simulink library "sm_testrig_common_gear_lib"  (R2021b)
settings: Solver=VariableStepAuto  StartTime=0.0  StopTime=10.0  RelTol=1e-3
values from neighbouring files (symbols this model uses):
  N = 10    [sm_extr_data_gear.m]
undefined symbols (not defined in the file or in its folder): b_gear_pd_asy, b_visc_frict_asy, f_gear_ad, f_gear_clr, f_gear_dd, f_gear_nt, f_gear_pd_asy, f_gear_rho, f_gear_rht, f_gear_th, f_mark_angle_range, f_mark_color, f_mark_radius_range, f_visc_frict_asy, X, Y, Z
libraries: sm_lib x8
settings Model: Creator=The MathWorks, Inc.  LastModifiedBy=The MathWorks, Inc.
settings SolverCC: AlgebraicLoopSolver=TrustRegion
settings DataIOCC: ReturnWorkspaceOutputs=off
settings DebuggingCC: SFMachineParentedDataDiag=warning  ArithmeticOperatorsInVariantConditions=warning
settings SFSimCC: SimUseLocalCustomCode=off  CustomCodeUndefinedFunction=UseInterfaceOnly
settings RTWCC: RTWUseLocalCustomCode=off

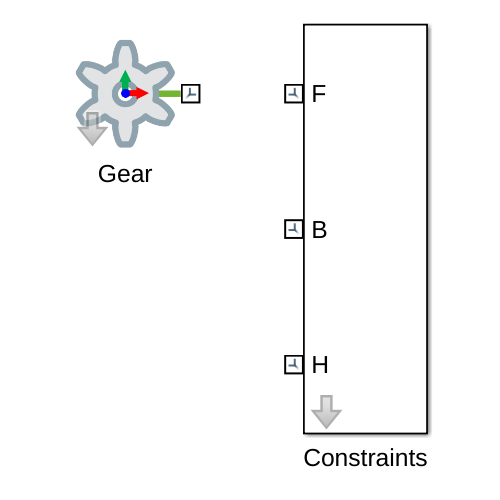
[thumbnail: Simulink's stored preview of the top-level diagram]
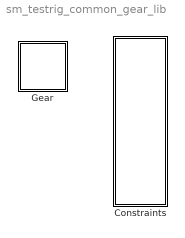
== system sm_testrig_common_gear_lib ==
  Constraints : Subsystem  mask(Common Gear Assembly Constraints){popup_gear_type=External, b_gear_pd=b_gear_pd_asy, f_gear_pd=f_gear_pd_asy, b_visc_frict=b_visc_frict_asy, f_visc_frict=f_visc_frict_asy}
      mask prompts: popup_gear_type "Gear Type"
      mask help: Model connects all required constraints for a common gear assembly. Contains two Revolute Joints and a Common Gear Constraint, all oriented and positioned according to the Common Gear Constraint requirements.
      mask init:
      | gear_constr_type = get_param(gcb,'popup_gear_type');
      | set_param([gcb '/Common Gear Constraint'],'GearType',gear_constr_type);
      | if(strcmpi(gear_constr_type,'External'))
      |     gear_axis_offset = (f_gear_pd+b_gear_pd)/2;
      | else
      |     gear_axis_offset = (f_gear_pd-b_gear_pd)/2;
      | end
      mask TypeOptions popup_gear_type: External | Internal
      mask DialogControl Control3 Prompt: Gear B
      mask DialogControl Control4 Prompt: Gear F
      mask DialogControl Control5 Prompt: Pitch Diameter (m)
      mask DialogControl Control6 Prompt: Bearing Friction N*m/(deg/s)
  Gear : Subsystem  mask(Gear){popup_gear_type=External, gear_pd=f_gear_pd_asy, gear_nt=f_gear_nt, gear_th=f_gear_th, gear_rh=f_gear_rht, gear_rt=f_gear_rht, gear_rho=f_gear_rho, gear_clr=f_gear_clr, popup_ad_dd=Default, gear_ad=f_gear_ad, gear_dd=f_gear_dd, popup_markings=Two, mark_radius_range=f_mark_radius_range, mark_angle_range=f_mark_angle_range, mark_color=f_mark_color}
      mask prompts: popup_gear_type "Gear Type"; gear_pd "Pitch Diameter (m)"; gear_nt "Number of Teeth"; gear_th "Gear Thickness (m)"; gear_rh "Hole Radius (m)"; gear_rt "Outer Radius (m)"; gear_rho "Density (kg/m^3)"; gear_clr "Color [RGB]"; popup_ad_dd "Addendum, Dedendum"; gear_ad "Addendum (m)"; gear_dd "Dedendum (m)"; popup_markings "Show Markings"; mark_radius_range "Radial Range [min max] (0-1)"; mark_angle_range "Sweep Angle [0-180] (deg)"; mark_color "Color [RGB]"
      mask help: This block models an external or internal involute tooth gear. The gear tooth profile assumes a pressure angle of 14.5 degrees.
      mask init:
      | if (strcmp(get_param(gcb,'popup_gear_type'),'External'))
      |     gear_holeORouter = gear_rh;
      | else
      |     gear_holeORouter = gear_rt;
      | end
      | 
      | if (strcmp(get_param(gcb,'popup_ad_dd'),'Default'))
      | gear_xsec = sm_extr_data_gear(...
      |     get_param(gcb,'popup_gear_type'),...
      |     gear_pd, gear_nt, gear_holeORouter);
      | else
      | gear_xsec = sm_extr_data_gear(...
      |     get_param(gcb,'popup_gear_type'),...
      |     gear_pd, gear_nt, gear_holeORouter, gear_ad, gear_dd);
      | end
      | 
      | mark_xsec =  [
      |     gear_pd/2*max(mark_radius_range) gear_th/1.9; 
      |     gear_pd/2*min(mark_radius_range) gear_th/1.9; 
      |     gear_pd/2*min(mark_radius_range) -gear_th/1.9; 
      |     gear_pd/2*max(mark_radius_range) -gear_th/1.9];
      | 
      | mark_1_opc = 0;
      | mark_2_opc = 0;
      | 
      | if(popup_markings == 2)
      |     mark_1_opc = 1;
      | elseif(popup_markings == 3)
      |     mark_1_opc = 1;
      |     mark_2_opc = 1;
      | end
      mask TypeOptions popup_gear_type: External | Internal
      mask Callback popup_gear_type:
      | maskObj = Simulink.Mask.get(gcb);
      | grh_h = maskObj.getParameter('gear_rh');
      | grt_h = maskObj.getParameter('gear_rt');
      | if strcmp(get_param(gcb,'popup_gear_type'),'External')
      |     grh_h.Visible = 'on';
      |     grt_h.Visible = 'off';
      | else
      |     grh_h.Visible = 'off';
      |     grt_h.Visible = 'on';
      | end
      | clear maskObj grh_h grt_h
      mask TypeOptions popup_ad_dd: Default | Specify
      mask Callback popup_ad_dd:
      | maskObj = Simulink.Mask.get(gcb);
      | gad_h = maskObj.getParameter('gear_ad');
      | gdd_h = maskObj.getParameter('gear_dd');
      | if strcmp(get_param(gcb,'popup_ad_dd'),'Default')
      |     gad_h.Visible = 'off';
      |     gdd_h.Visible = 'off';
      | else
      |     gad_h.Visible = 'on';
      |     gdd_h.Visible = 'on';
      | end
      | clear maskObj gad_h gdd_h
      mask TypeOptions popup_markings: None | One | Two
      mask Callback popup_markings:
      | maskObj = Simulink.Mask.get(gcb);
      | mkc_h = maskObj.getDialogControl('container_markings');
      | if strcmp(get_param(gcb,'popup_markings'),'None')
      |     mkc_h.Visible = 'off';
      | else
      |     mkc_h.Visible = 'on';
      | end
      | clear maskObj mkc_h
      mask DialogControl Control2 Prompt: Plot Profile
      mask DialogControl Control2 Callback:
      | v = get_param(gcb,'MaskWSVariables');
      | getMaskValue = containers.Map({v.Name}',{v.Value}');
      | 
      | if (strcmp(get_param(gcb,'popup_gear_type'),'External'))
      |     gear_holeORouter = getMaskValue('gear_rh');
      | else
      |     gear_holeORouter = getMaskValue('gear_rt');
      | end
      | 
      | if (strcmp(get_param(gcb,'popup_ad_dd'),'Default'))
      |     evalin('base',...
      |         sprintf('Extr_Data_Gear(''%s'',%s,%s,%s,''%s'');',...
      |         get_param(gcb,'popup_gear_type'),...
      |         num2str(getMaskValue('gear_pd')),...
      |         num2str(getMaskValue('gear_nt')),...
      |         num2str(gear_holeORouter),'plot'));
      | else
      |     evalin('base',...
      |         sprintf('Extr_Data_Gear(''%s'',%s,%s,%s,%s,%s,''%s'');',...
      |         get_param(gcb,'popup_gear_type'),...
      |         num2str(getMaskValue('gear_pd')),...
      |         num2str(getMaskValue('gear_nt')),...
      |         num2str(gear_holeORouter),...
      |         num2str(getMaskValue('gear_ad')),...
      |         num2str(getMaskValue('gear_dd')),'plot'));
      | end
      mask Display:
      | if(strcmpi(get_param(gcb,'popup_gear_type'),'Internal'))
      |     image('sm_testrig_common_gear_internal_gear.png');
      | else
      |     image('sm_testrig_common_gear_external_gear.png');
      | end

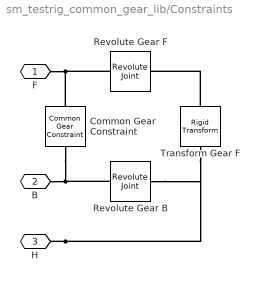
== system sm_testrig_common_gear_lib/Constraints ==
  Common Gear Constraint : sm_lib/Gears and Couplings/Gears/Common Gear Constraint  GearType=External  SpecificationType=PitchCircleRadii  CenterDistance=30  CenterDistanceUnits=cm  GearRatio=0.5  BaseGearRadius=b_gear_pd/2  BaseGearRadiusUnits=m  FollGearRadius=f_gear_pd/2  FollGearRadiusUnits=m  AssemblyGearRotation=Free
      settings: SourceProductBaseCode=MS
  Revolute Gear B : sm_lib/Joints/Revolute Joint  JointMode=Normal  SenseConstraintForce=off  SenseConstraintForceX=off  SenseConstraintForceY=off  SenseConstraintForceZ=off  SenseConstraintTorque=off  SenseConstraintTorqueX=off  SenseConstraintTorqueY=off  SenseConstraintTorqueZ=off  SenseTotalForce=off  SenseTotalForceX=off  SenseTotalForceY=off  SenseTotalForceZ=off  SenseTotalTorque=off  SenseTotalTorqueX=off  SenseTotalTorqueY=off  SenseTotalTorqueZ=off  CompositeWrenchDir=FollowerOnBase  CompositeWrenchFrame=BaseFrame  EquilibriumPosition=0  EquilibriumPositionUnits=deg  SpringStiffness=0  SpringStiffnessUnits=N*m/deg  DampingCoefficient=b_visc_frict  DampingCoefficientUnits=N*m/(deg/s)  TorqueActuationMode=NoTorque  MotionActuationMode=ComputedMotion  SensePosition=off  SenseVelocity=off  SenseAcceleration=off  SenseTorqueForce=off  SenseLowerLimitTorqueForce=off  SenseUpperLimitTorqueForce=off  LowerLimitSpecify=off  LowerLimitBound=-90  LowerLimitBoundUnits=deg  LowerLimitStiffness=1e4  LowerLimitStiffnessUnits=N*m/deg  LowerLimitDamping=10  LowerLimitDampingUnits=N*m/(deg/s)  LowerLimitTransitionRegionWidth=0.1  LowerLimitTransitionRegionWidthUnits=deg  UpperLimitSpecify=off  UpperLimitBound=90  UpperLimitBoundUnits=deg  UpperLimitStiffness=1e4  UpperLimitStiffnessUnits=N*m/deg  UpperLimitDamping=10  UpperLimitDampingUnits=N*m/(deg/s)  UpperLimitTransitionRegionWidth=0.1  UpperLimitTransitionRegionWidthUnits=deg  PositionTargetSpecify=off  PositionTargetPriority=High  PositionTargetValue=0  PositionTargetValueUnits=deg  VelocityTargetSpecify=off  VelocityTargetPriority=High  VelocityTargetValue=0  VelocityTargetValueUnits=deg/s
  Revolute Gear F : sm_lib/Joints/Revolute Joint  JointMode=Normal  SenseConstraintForce=off  SenseConstraintForceX=off  SenseConstraintForceY=off  SenseConstraintForceZ=off  SenseConstraintTorque=off  SenseConstraintTorqueX=off  SenseConstraintTorqueY=off  SenseConstraintTorqueZ=off  SenseTotalForce=off  SenseTotalForceX=off  SenseTotalForceY=off  SenseTotalForceZ=off  SenseTotalTorque=off  SenseTotalTorqueX=off  SenseTotalTorqueY=off  SenseTotalTorqueZ=off  CompositeWrenchDir=FollowerOnBase  CompositeWrenchFrame=BaseFrame  EquilibriumPosition=0  EquilibriumPositionUnits=deg  SpringStiffness=0  SpringStiffnessUnits=N*m/deg  DampingCoefficient=f_visc_frict  DampingCoefficientUnits=N*m/(deg/s)  TorqueActuationMode=NoTorque  MotionActuationMode=ComputedMotion  SensePosition=off  SenseVelocity=off  SenseAcceleration=off  SenseTorqueForce=off  SenseLowerLimitTorqueForce=off  SenseUpperLimitTorqueForce=off  LowerLimitSpecify=off  LowerLimitBound=-90  LowerLimitBoundUnits=deg  LowerLimitStiffness=1e4  LowerLimitStiffnessUnits=N*m/deg  LowerLimitDamping=10  LowerLimitDampingUnits=N*m/(deg/s)  LowerLimitTransitionRegionWidth=0.1  LowerLimitTransitionRegionWidthUnits=deg  UpperLimitSpecify=off  UpperLimitBound=90  UpperLimitBoundUnits=deg  UpperLimitStiffness=1e4  UpperLimitStiffnessUnits=N*m/deg  UpperLimitDamping=10  UpperLimitDampingUnits=N*m/(deg/s)  UpperLimitTransitionRegionWidth=0.1  UpperLimitTransitionRegionWidthUnits=deg  PositionTargetSpecify=on  PositionTargetPriority=High  PositionTargetValue=45  PositionTargetValueUnits=deg  VelocityTargetSpecify=off  VelocityTargetPriority=High  VelocityTargetValue=0  VelocityTargetValueUnits=deg/s
  Transform Gear F : sm_lib/Frames and Transforms/Rigid Transform  TranslationMethod=StandardAxis  TranslationStandardOffset=gear_axis_offset  TranslationLengthUnit=m  TranslationStandardAxis=+X  TranslationCartesianOffset=[0 0 0]  TranslationROffset=0  TranslationROffsetUnits=m  TranslationZOffset=0  TranslationZOffsetUnits=m  TranslationThetaOffset=0  TranslationThetaOffsetUnits=deg  RotationMethod=None  RotationAngleUnits=deg  RotationStandardAxis=+Z  RotationAngle=0  RotationArbitraryAxis=[0 0 1]  FollAlignAxisA=+X  BaseAlignAxisA=+Y  FollAlignAxisB=+Y  BaseAlignAxisB=+Z  RotationSequenceAxes=FollowerAxes  RotationSequence=XYX  RotationSequenceAngles=[0 0 0]  RotationSequenceAnglesUnits=deg  RotationMatrix=[1 0 0; 0 1 0; 0 0 1]
  F : PMIOPort  Side=Left
  B : PMIOPort  Port=2  Side=Left
  H : PMIOPort  Port=3  Side=Left
  connections:
  Revolute Gear B/RConn1 -- Common Gear Constraint/LConn1 -- B/RConn1
  Revolute Gear F/RConn1 -- Common Gear Constraint/RConn1 -- F/RConn1
  Transform Gear F/RConn1 -- Revolute Gear F/LConn1
  H/RConn1 -- Transform Gear F/LConn1 -- Revolute Gear B/LConn1

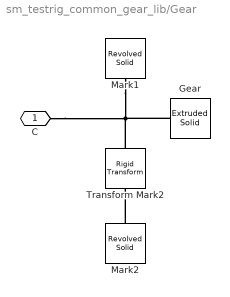
== system sm_testrig_common_gear_lib/Gear ==
  Gear : sm_lib/Body Elements/Extruded Solid  GraphicAmbientColor=[0.15 0.15 0.15 1.0]  BasedOnType=Density  CenterOfMass=[0 0 0]  CenterOfMassUnits=m  GraphicDiffuseColor=gear_clr  ExportConvexHullGeometry=off  ExtrusionCrossSection=gear_xsec  ExtrusionCrossSectionUnits=m  Density=gear_rho  DensityUnits=kg/(m^3)  DoExposeReferenceFrame=on  GraphicEmissiveColor=[0.0 0.0 0.0 1.0]  ExportEntireGeometry=off  ExtrusionLength=gear_th  ExtrusionLengthUnits=m  ExtrusionType=General  SerializedFrames=<Frames/>  MarkerShape=Sphere  MarkerSize=10  GraphicType=FromGeometry  InertiaType=CalculateFromGeometry  Mass=1  MassUnits=kg  MomentsOfInertia=[1 1 1]  MomentsOfInertiaUnits=kg*m^2  PolygonNumSides=3  GraphicOpacity=1.0  PolygonOuterRadius=1  PolygonOuterRadiusUnits=m  ProductsOfInertia=[0 0 0]  ProductsOfInertiaUnits=kg*m^2  GraphicShininess=75  GraphicSpecularColor=[0.5 0.5 0.5 1.0]  GraphicVisPropType=SimpleVisualProperties
  Mark1 : sm_lib/Body Elements/Revolved Solid  GraphicAmbientColor=[0.15 0.15 0.15 1.0]  BasedOnType=Density  CenterOfMass=[0 0 0]  CenterOfMassUnits=m  GraphicDiffuseColor=mark_color  ExportConvexHullGeometry=off  Density=0  DensityUnits=kg/m^3  DoExposeReferenceFrame=on  GraphicEmissiveColor=[0.0 0.0 0.0 1.0]  ExportEntireGeometry=off  SerializedFrames=<Frames/>  MarkerShape=Sphere  MarkerSize=10  GraphicType=FromGeometry  InertiaType=CalculateFromGeometry  Mass=1  MassUnits=kg  MomentsOfInertia=[1 1 1]  MomentsOfInertiaUnits=kg*m^2  GraphicOpacity=mark_1_opc  ProductsOfInertia=[1 1 1]  ProductsOfInertiaUnits=kg*m^2  RevolutionCrossSection=mark_xsec  RevolutionCrossSectionUnits=m  RevolutionAngle=mark_angle_range  RevolutionAngleUnits=deg  RevolutionExtent=Custom  GraphicShininess=75  GraphicSpecularColor=[0.5 0.5 0.5 1.0]  GraphicVisPropType=SimpleVisualProperties
  Mark2 : sm_lib/Body Elements/Revolved Solid  GraphicAmbientColor=[0.15 0.15 0.15 1.0]  BasedOnType=Density  CenterOfMass=[0 0 0]  CenterOfMassUnits=m  GraphicDiffuseColor=mark_color  ExportConvexHullGeometry=off  Density=0  DensityUnits=kg/m^3  DoExposeReferenceFrame=on  GraphicEmissiveColor=[0.0 0.0 0.0 1.0]  ExportEntireGeometry=off  SerializedFrames=<Frames/>  MarkerShape=Sphere  MarkerSize=10  GraphicType=FromGeometry  InertiaType=CalculateFromGeometry  Mass=1  MassUnits=kg  MomentsOfInertia=[1 1 1]  MomentsOfInertiaUnits=kg*m^2  GraphicOpacity=mark_2_opc  ProductsOfInertia=[1 1 1]  ProductsOfInertiaUnits=kg*m^2  RevolutionCrossSection=mark_xsec  RevolutionCrossSectionUnits=m  RevolutionAngle=mark_angle_range  RevolutionAngleUnits=deg  RevolutionExtent=Custom  GraphicShininess=75  GraphicSpecularColor=[0.5 0.5 0.5 1.0]  GraphicVisPropType=SimpleVisualProperties
  Transform Mark2 : sm_lib/Frames and Transforms/Rigid Transform  TranslationMethod=None  TranslationStandardOffset=0  TranslationLengthUnit=m  TranslationStandardAxis=+Z  TranslationCartesianOffset=[0 0 0]  TranslationROffset=0  TranslationROffsetUnits=m  TranslationZOffset=0  TranslationZOffsetUnits=m  TranslationThetaOffset=0  TranslationThetaOffsetUnits=deg  RotationMethod=StandardAxis  RotationAngleUnits=deg  RotationStandardAxis=+Y  RotationAngle=180  RotationArbitraryAxis=[0 0 1]  FollAlignAxisA=+X  BaseAlignAxisA=+Y  FollAlignAxisB=+Y  BaseAlignAxisB=+Z  RotationSequenceAxes=FollowerAxes  RotationSequence=XYX  RotationSequenceAngles=[0 0 0]  RotationSequenceAnglesUnits=deg  RotationMatrix=[1 0 0; 0 1 0; 0 0 1]
  C : PMIOPort  Side=Right
  connections:
  Mark2/RConn1 -- Transform Mark2/RConn1
  Mark1/RConn1 -- Gear/RConn1 -- Transform Mark2/LConn1 -- C/RConn1
